simulink model "Reusable_NonReusable"  (R2024a)
settings: Solver=FixedStepDiscrete  StartTime=0.0  StopTime=10.0  FixedStep=1  RelTol=1e-3
model workspace (MAT data in the model file):
  Kp = Simulink.Parameter
  Kp.Value = 5
  Kp.Complexity = 'real'
  Kp.Dimensions = [1 1]
  Kp.DataType = 'uint8'
settings Model: Creator=BIDO  LastModifiedBy=BIDO
settings OptimizationCC: UseDivisionForNetSlopeComputation=on  GainParamInheritBuiltInType=on  UseFloatMulNetSlope=on  PassReuseOutputArgsAs=Individual arguments  ZeroExternalMemoryAtStartup=off  ZeroInternalMemoryAtStartup=off  InitFltsAndDblsToZero=on  NoFixptDivByZeroProtection=on  EfficientFloat2IntCast=on  LifeSpan=1  OptimizeBlockOrder=speed  DifferentSizesBufferReuse=on  EfficientTunableParamExpr=on
settings DebuggingCC: ParameterTunabilityLossMsg=error
settings HardwareCC: ProdLongLongMode=on
settings SFSimCC: MATLABDynamicMemAlloc=off
settings RTWCC: Description=Embedded Coder  SystemTargetFile=ert.tlc  TemplateMakefile=ert_default_tmf
settings CodeAppCC: ForceParamTrailComments=on  IgnoreCustomStorageClasses=off  OperatorAnnotations=on  SimulinkDataObjDesc=on  SFDataObjDesc=on  CustomSymbolStrGlobalVar=rt$N$M  CustomSymbolStrType=$N$M  CustomSymbolStrFcn=$N$M$F  CustomSymbolStrMacro=$N$M  InsertBlockDesc=on
settings ERTTargetCC: TargetLangStandard=C99 (ISO)  GenerateSampleERTMain=on  IncludeMdlTerminateFcn=off  CombineSignalStateStructs=on  SuppressErrorStatus=on  SupportAbsoluteTime=off  SupportComplex=off  RootIOFormat=Part of model data structure  ERTCustomFileTemplate=example_file_process.tlc  ERTFilePackagingFormat=CompactWithDataFile

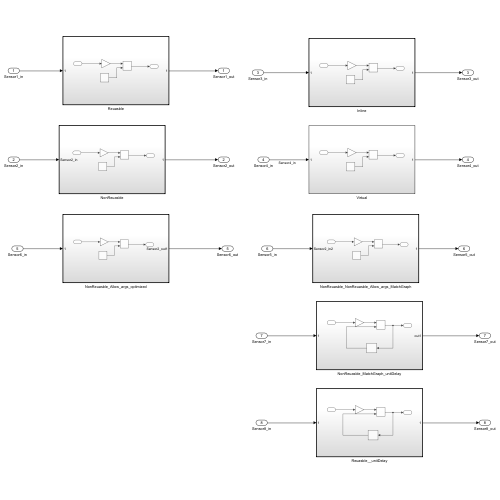
[thumbnail: Simulink's stored preview of the top-level diagram]
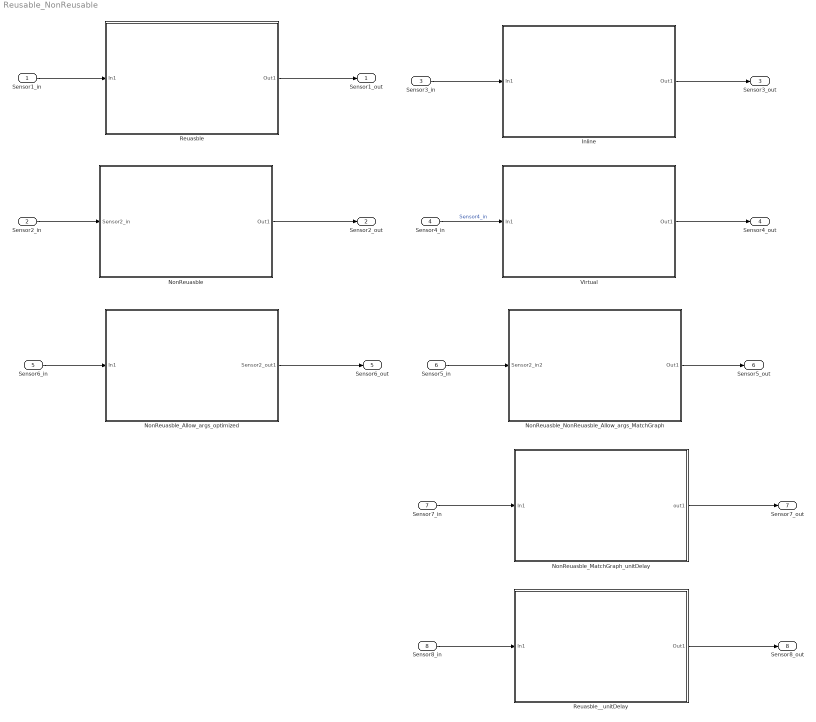
== system Reusable_NonReusable ==
  Sensor1_in : Inport
  Sensor2_in : Inport  Port=2
  Sensor3_in : Inport  Port=3
  Sensor4_in : Inport  Port=4
  Sensor6_in : Inport  Port=5
  Sensor5_in : Inport  Port=6
  Sensor7_in : Inport  Port=7
  Sensor8_in : Inport  Port=8
  Inline : Subsystem  TreatAsAtomicUnit=on
      settings: RTWSystemCode=Inline  RTWFcnNameOpts=Use subsystem name  RTWFileNameOpts=Use subsystem name
  NonReuasble : Subsystem  TreatAsAtomicUnit=on
      settings: RTWSystemCode=Nonreusable function  RTWFcnNameOpts=Use subsystem name
  NonReuasble_Allow_args_optimized : Subsystem  TreatAsAtomicUnit=on
      settings: RTWSystemCode=Nonreusable function  RTWFcnNameOpts=Use subsystem name  FunctionInterfaceSpec=Allow arguments (Optimized)
  NonReuasble_MatchGraph_unitDelay : Subsystem  TreatAsAtomicUnit=on
      settings: RTWSystemCode=Nonreusable function  RTWFcnNameOpts=Use subsystem name  FunctionInterfaceSpec=Allow arguments (Optimized)
  NonReuasble_NonReuasble_Allow_args_MatchGraph : Subsystem  TreatAsAtomicUnit=on
      settings: RTWSystemCode=Nonreusable function  RTWFcnNameOpts=Use subsystem name  FunctionInterfaceSpec=Allow arguments (Optimized)
  Reuasble : Subsystem  TreatAsAtomicUnit=on
      settings: RTWFcnNameOpts=Use subsystem name
  Reuasble__unitDelay : Subsystem  TreatAsAtomicUnit=on
      settings: RTWFcnNameOpts=Use subsystem name  FunctionInterfaceSpec=Allow arguments (Match graphical interface)
  Virtual : Subsystem
      settings: RTWSystemCode=Nonreusable function  RTWFcnNameOpts=Use subsystem name  RTWFileNameOpts=Use subsystem name
  Sensor1_out : Outport
  Sensor2_out : Outport  Port=2
  Sensor3_out : Outport  Port=3
  Sensor4_out : Outport  Port=4
  Sensor6_out : Outport  Port=5
  Sensor5_out : Outport  Port=6
  Sensor7_out : Outport  Port=7
  Sensor8_out : Outport  Port=8
  wires:
  Sensor1_in/1 -> Reuasble/1(In1)
  Reuasble/1(Out1) -> Sensor1_out/1
  NonReuasble/1(Out1) -> Sensor2_out/1
  Inline/1(Out1) -> Sensor3_out/1
  Sensor3_in/1 -> Inline/1(In1)
  Sensor4_in/1 -> Virtual/1(In1)  "Sensor4_in"
  Virtual/1(Out1) -> Sensor4_out/1
  Sensor5_in/1 -> NonReuasble_NonReuasble_Allow_args_MatchGraph/1(Sensor2_in2)
  Sensor8_in/1 -> Reuasble__unitDelay/1(In1)
  Sensor2_in/1 -> NonReuasble/1(Sensor2_in)
  Sensor6_in/1 -> NonReuasble_Allow_args_optimized/1(In1)
  NonReuasble_NonReuasble_Allow_args_MatchGraph/1(Out1) -> Sensor5_out/1
  NonReuasble_Allow_args_optimized/1(Sensor2_out1) -> Sensor6_out/1
  Reuasble__unitDelay/1(Out1) -> Sensor8_out/1
  Sensor7_in/1 -> NonReuasble_MatchGraph_unitDelay/1(In1)
  NonReuasble_MatchGraph_unitDelay/1(out1) -> Sensor7_out/1

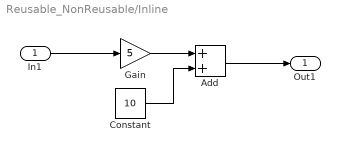
== system Reusable_NonReusable/Inline ==
  In1 : Inport
  Add : Sum
  Constant : Constant  Value=10
  Gain : Gain  Gain=5
  Out1 : Outport
  wires:
  Add/1 -> Out1/1
  Constant/1 -> Add/2
  In1/1 -> Gain/1
  Gain/1 -> Add/1

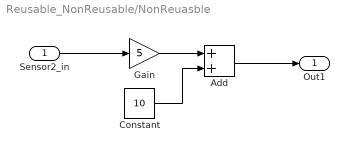
== system Reusable_NonReusable/NonReuasble ==
  Sensor2_in : Inport
  Add : Sum
  Constant : Constant  Value=10
  Gain : Gain  Gain=5
  Out1 : Outport
  wires:
  Add/1 -> Out1/1
  Constant/1 -> Add/2
  Sensor2_in/1 -> Gain/1
  Gain/1 -> Add/1

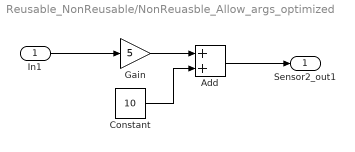
== system Reusable_NonReusable/NonReuasble_Allow_args_optimized ==
  In1 : Inport
  Add : Sum
  Constant : Constant  Value=10
  Gain : Gain  Gain=5
  Sensor2_out1 : Outport
  wires:
  Gain/1 -> Add/1
  In1/1 -> Gain/1
  Constant/1 -> Add/2
  Add/1 -> Sensor2_out1/1

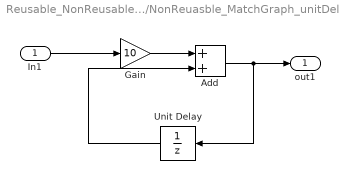
== system Reusable_NonReusable/NonReuasble_MatchGraph_unitDelay ==
  In1 : Inport
  Add : Sum
  Gain : Gain  Gain=10
  Unit Delay : UnitDelay  SampleTime=-1  HasFrameUpgradeWarning=on
  out1 : Outport
  wires:
  Gain/1 -> Add/1
  In1/1 -> Gain/1
  Unit Delay/1 -> Add/2
  Add/1 -> Unit Delay/1, out1/1

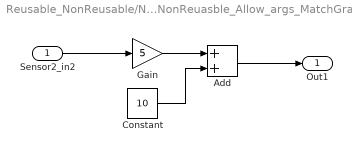
== system Reusable_NonReusable/NonReuasble_NonReuasble_Allow_args_MatchGraph ==
  Sensor2_in2 : Inport
  Add : Sum
  Constant : Constant  Value=10
  Gain : Gain  Gain=5
  Out1 : Outport
  wires:
  Add/1 -> Out1/1
  Constant/1 -> Add/2
  Sensor2_in2/1 -> Gain/1
  Gain/1 -> Add/1

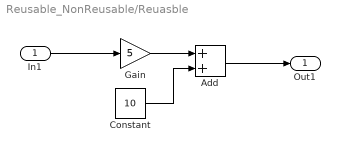
== system Reusable_NonReusable/Reuasble ==
  In1 : Inport
  Add : Sum
  Constant : Constant  Value=10
  Gain : Gain  Gain=5
  Out1 : Outport
  wires:
  Gain/1 -> Add/1
  In1/1 -> Gain/1
  Constant/1 -> Add/2
  Add/1 -> Out1/1

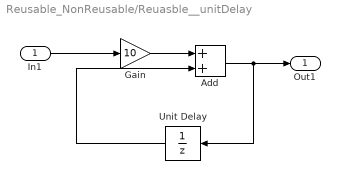
== system Reusable_NonReusable/Reuasble__unitDelay ==
  In1 : Inport
  Add : Sum
  Gain : Gain  Gain=10
  Unit Delay : UnitDelay  SampleTime=-1  HasFrameUpgradeWarning=on
  Out1 : Outport
  wires:
  Add/1 -> Out1/1, Unit Delay/1
  Unit Delay/1 -> Add/2
  In1/1 -> Gain/1
  Gain/1 -> Add/1

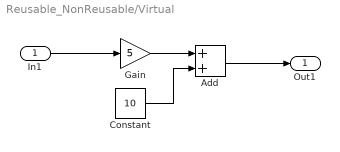
== system Reusable_NonReusable/Virtual ==
  In1 : Inport
  Add : Sum
  Constant : Constant  Value=10
  Gain : Gain  Gain=5
  Out1 : Outport
  wires:
  Gain/1 -> Add/1
  In1/1 -> Gain/1
  Constant/1 -> Add/2
  Add/1 -> Out1/1
